simulink model "statespacemodel_48to200V"  (R2026a)
settings: Solver=VariableStepAuto  StopTime=0.2
settings Model: Creator=aisik  LastModifiedBy=aisik

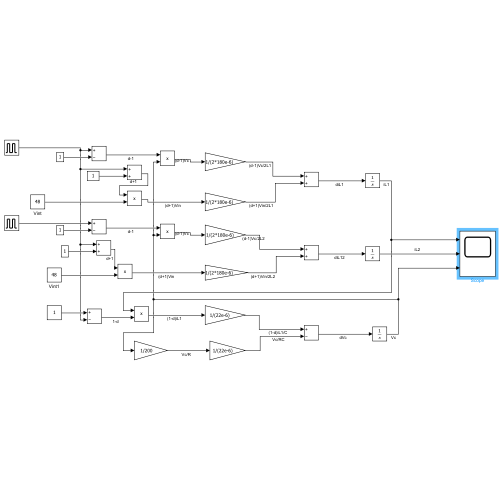
[thumbnail: Simulink's stored preview of the top-level diagram]
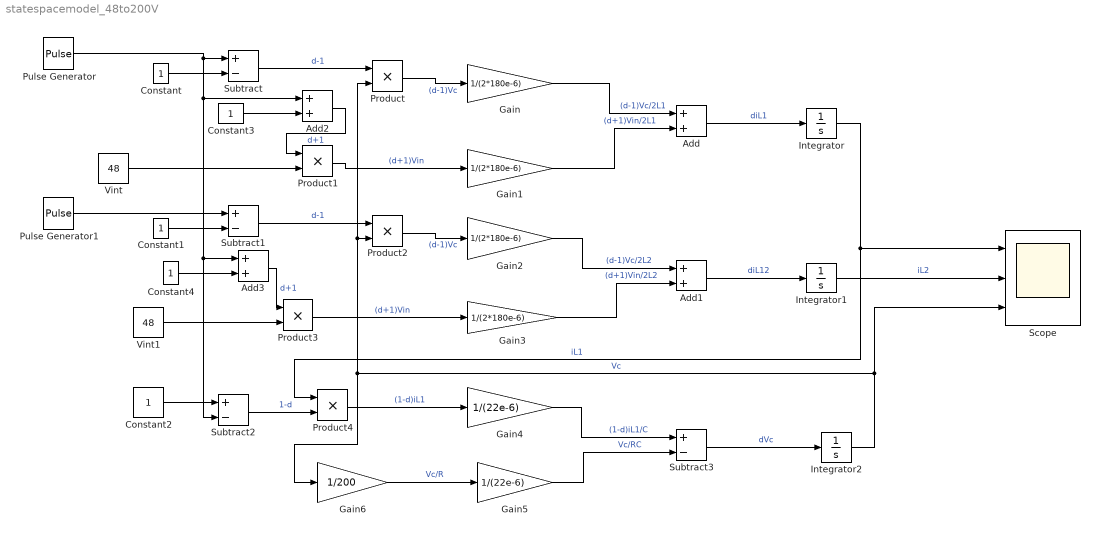
== system statespacemodel_48to200V ==
  Add{,1..3} (4 alike) : Sum
  Constant{,1..4} (5 alike) : Constant
  Gain{,1..3} (4 alike) : Gain  Gain=1/(2*180e-6)
  Gain4 : Gain  Gain=1/(22e-6)
  Gain5 : Gain  Gain=1/(22e-6)
  Gain6 : Gain  Gain=1/200
  Integrator : Integrator
  Integrator1 : Integrator
  Integrator2 : Integrator
  Product{,1..4} (5 alike) : Product
  Pulse Generator : DiscretePulseGenerator  PulseType=Time based  Period=1/(50e3)  PulseWidth=0.61*100
  Pulse Generator1 : DiscretePulseGenerator  PulseType=Time based  Period=1/50e3  PulseWidth=0.61*100
  Scope : Scope  NumInputPorts=3
      settings: ActiveDisplayYMinimum=-54.090090121632379  ActiveDisplayYMaximum=62.856228903972735
  Subtract{,1..3} (4 alike) : Sum  Inputs=+-
  Vint : Constant  Value=48
  Vint1 : Constant  Value=48
  wires:
  Pulse Generator/1 -> Subtract2/2, Add3/1, Add2/1, Subtract/1
  Constant/1 -> Subtract/2
  Subtract/1 -> Product/1  "d-1"
  Product/1 -> Gain/1  "(d-1)Vc"
  Product1/1 -> Gain1/1  "(d+1)Vin"
  Gain/1 -> Add/1  "(d-1)Vc/2L1"
  Gain1/1 -> Add/2  "(d+1)Vin/2L1"
  Add/1 -> Integrator/1  "diL1"
  Integrator/1 -> Product4/1, Scope/1  "iL1"
  Product2/1 -> Gain2/1  "(d-1)Vc"
  Product3/1 -> Gain3/1  "(d+1)Vin"
  Constant1/1 -> Subtract1/2
  Pulse Generator1/1 -> Subtract1/1
  Gain2/1 -> Add1/1  "(d-1)Vc/2L2"
  Subtract1/1 -> Product2/1  "d-1"
  Add1/1 -> Integrator1/1  "diL12"
  Integrator1/1 -> Scope/2  "iL2"
  Gain3/1 -> Add1/2  "(d+1)Vin/2L2"
  Vint1/1 -> Product3/2
  Constant2/1 -> Subtract2/1
  Subtract2/1 -> Product4/2  "1-d"
  Product4/1 -> Gain4/1  "(1-d)iL1"
  Gain6/1 -> Gain5/1  "Vc/R"
  Gain5/1 -> Subtract3/2  "Vc/RC"
  Gain4/1 -> Subtract3/1  "(1-d)iL1/C"
  Subtract3/1 -> Integrator2/1  "dVc"
  Integrator2/1 -> Scope/3, Gain6/1, Product/2, Product2/2  "Vc"
  Constant3/1 -> Add2/2
  Add2/1 -> Product1/1  "d+1"
  Vint/1 -> Product1/2
  Constant4/1 -> Add3/2
  Add3/1 -> Product3/1  "d+1"
